simulink model "Vehicle_Model_Controller_2018"  (R2020a)
settings: Solver=FixedStepAuto  StartTime=0.0  StopTime=60  FixedStep=0.015  MaxStep=0.1  RelTol=1e-3
model workspace (MAT data in the model file):
  Kp = 10
  understeer_gradient = 0.05
undefined symbols (not defined in the file or in its folder): front_forces, rear_forces
libraries: fl_lib x24, nesl_utility x20, sdl_lib x8, simulink x1, vehdynlibsteering x1, autolibshared x1, autolibdatasheetbattery x1
(part 2 of 2)

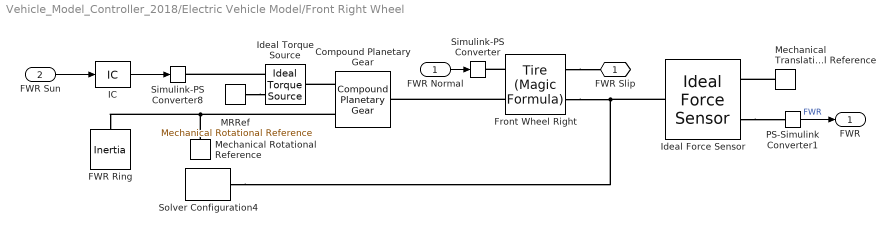
== system Vehicle_Model_Controller_2018/Electric Vehicle Model/Front Right Wheel ==
  FWR Normal : Inport
  FWR Sun : Inport  Port=2
  Compound Planetary Gear : sdl_lib/Gears/Compound Planetary Gear  rp_ratio=84/23  ps_ratio=37/24  friction_model=sdl.enum.gear_friction.none  mu_visc=[0, 0] N*m/(rad/s)  efficiency=[.96, .98]  temperature_TLU=[280, 300, 320] K  efficiency_sp_TLU=[.95, .9, .85]  efficiency_rp_TLU=[.95, .9, .85]  pwr_thr=[.001, .001] W  thermal_mass=50 J/K  T_init=300 K  model_inertia=simscape.enum.onoff.off  planet_inertia=0.001 kg*m^2
      settings: SourceProductBaseCode=LD  InternalSimscapePortConfiguration="{\"Bottom\":[],\"Left\":[{\"id\":\"C\",\"label\":\"C\",\"type\":\"foundation.mechanical.rotational.rotational\"}],\"Right\":[{\"id\":\"R\",\"label\":\"R\",\"type\":\"foundation.mechanical.rotational.rotational\"},{\"id\":\"S\",\"label\":\"S\",\"type\":\"foundation.mechanical.rotational.rotational\"}],\"Top\":[]}"
  FWR Ring : fl_lib/Mechanical/Rotational Elements/Inertia  inertia=0.1 kg*m^2  num_ports=foundation.enum.numPorts2.one  w_specify=off  w_priority=High  w=0 rad/s  w_nominal_specify=off  w_nominal_unit=rad/s  w_nominal_value=1  t_specify=off  t_priority=None  t=0 N*m  t_nominal_specify=off  t_nominal_unit=N*m  t_nominal_value=1
  Front Wheel Right : sdl_lib/Tires & Vehicles/Tire (Magic Formula)  parameterization=sdl.enum.magic_tire_model.peak  F_z1=3000 N  F_x1=3500 N  kappa1=10  B_m=10  C_m=1.9  D_m=1  E_m=0.97  fz0=4000 N  p_Cx=1.685  p_Dx=[1.21, -.037]  p_Ex=[.344, .095, -.02, 0]  p_Kx=[21.51, -.163, .245]  p_Hx=[-.002, .002]  p_Vx=[0, 0]  v_tr_thr=0.1 m/s  r_e=0.3 m  model_compliance=0  stiffness=2e5 N/m  damping=1000 N/(m/s)  model_inertia=0  inertia=0.03 kg*m^2  initial_velocity=0 rad/s  model_resistance=0  resistance_model=2  coeff=0.015  p_tire=250e3 Pa  alpha=-0.003  beta=0.97  coeff_a=84e-4  coeff_b=6.2e-4 s/m  coeff_c=1.6e-4 s^2/m^2  v_thr=0.001 m/s
  IC : InitialCondition  Value=0
  Ideal Force Sensor : fl_lib/Mechanical/Mechanical Sensors/Ideal Force Sensor
  Ideal Torque Source : fl_lib/Mechanical/Mechanical Sources/Ideal Torque Source
      settings: SourceProductName=Foundation Library
  MRRef : fl_lib/Mechanical/Rotational Elements/Mechanical Rotational Reference
      settings: SourceProductName=Foundation Library
  Mechanical Rotational Reference : fl_lib/Mechanical/Rotational Elements/Mechanical Rotational Reference
  Mechanical Translational Reference : fl_lib/Mechanical/Translational Elements/Mechanical Translational Reference
  PS-Simulink Converter1 : nesl_utility/PS-Simulink Converter  PhysicalDomain=network_engine_domain  SubClassName=ps_output  LeftPortType=input  RightPortType=output  PseudoPeriodic=off  Frequencies=[]  Unit=inherit  AffineConversion=off
      settings: SourceProductBaseCode=PW,SS
  Simulink-PS Converter : nesl_utility/Simulink-PS Converter  PhysicalDomain=network_engine_domain  SubClassName=ps_input  LeftPortType=input  RightPortType=output  PseudoPeriodic=off  Frequencies=[]  NoiseDistribution=none  NoiseParameters=[]  Unit=N  AffineConversion=off  FilteringAndDerivatives=zero  SimscapeFilterOrder=1  InputFilterTimeConstant=0.001  UdotUserProvided=0
      settings: SourceProductBaseCode=PW,SS
  Simulink-PS Converter8 : nesl_utility/Simulink-PS Converter  PhysicalDomain=network_engine_domain  SubClassName=ps_input  LeftPortType=input  RightPortType=output  PseudoPeriodic=off  Frequencies=[]  NoiseDistribution=none  NoiseParameters=[]  Unit=N*m  AffineConversion=off  FilteringAndDerivatives=zero  SimscapeFilterOrder=1  InputFilterTimeConstant=0.001  UdotUserProvided=0
      settings: SourceProductBaseCode=PW,SS
  Solver Configuration4 : nesl_utility/Solver Configuration  PhysicalDomain=network_engine_domain  SubClassName=solver  LeftPortType=input  RightPortType=generic  Tones=[]  Harmonics=[]  SimulateNoise=off  Profile=off  UseLocalSampling=off  EnableSwitchedLinearOptims=on  FrequencyDomain=off  UseCCode=off  RelTol=0.001  AbsTol=1e-06  MinStep=1e-09  ToWorkspace=off  RevertToSquareIcSolve=off  NumHomotopyIterations=100  PhasorMode=off  PhasorModeNumHarmonics=1  DoDC=on  ResidualTolerance=1e-09  UseLocalSolver=off  LocalSolverChoice=NE_BACKWARD_EULER_ADVANCER  LocalSolverSampleTime=0.001  DoFixedCost=off  MaxNonlinIter=3  MaxModeIter=2  ComputeImpulses=off  ImpulseIterations=2  LinearAlgebra=auto  EquationFormulation=NE_TIME_EF  DelaysMemoryBudget=1024  AutomaticFiltering=on  FilteringTimeConstant=0.001  PartitionStorageMethod=AS_NEEDED  PartitionMemoryBudget=1024  PartitionMethod=ROBUST
      settings: SourceProductBaseCode=PW,SS
  FWR Slip : PMIOPort  Side=Right
  FWR : Outport
  wires:
  PS-Simulink Converter1/1 -> FWR/1  "FWR"
  FWR Normal/1 -> Simulink-PS Converter/1
  IC/1 -> Simulink-PS Converter8/1
  FWR Sun/1 -> IC/1
  connections:
  Front Wheel Right/RConn1 -- FWR Slip/RConn1
  Front Wheel Right/LConn1 -- Simulink-PS Converter/RConn1
  Ideal Force Sensor/RConn2 -- PS-Simulink Converter1/LConn1
  Ideal Force Sensor/LConn1 -- Front Wheel Right/RConn2 -- Solver Configuration4/RConn1
  Mechanical Translational Reference/LConn1 -- Ideal Force Sensor/RConn1
  MRRef/LConn1 -- Ideal Torque Source/RConn2
  Compound Planetary Gear/RConn2 -- Ideal Torque Source/LConn1
  Ideal Torque Source/RConn1 -- Simulink-PS Converter8/RConn1
  Front Wheel Right/LConn2 -- Compound Planetary Gear/LConn1
  Mechanical Rotational Reference/LConn1 -- FWR Ring/LConn1 -- Compound Planetary Gear/RConn1

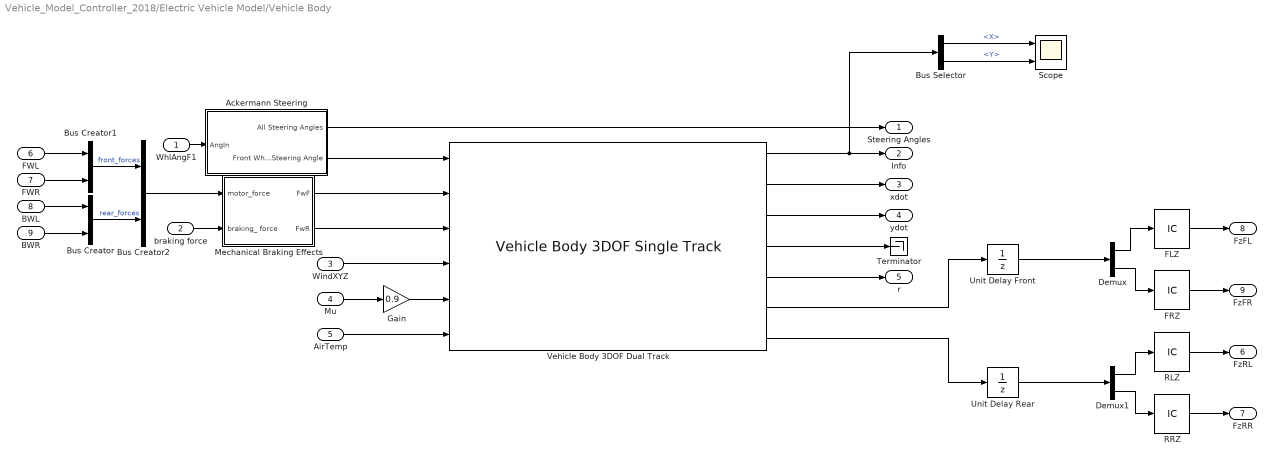
== system Vehicle_Model_Controller_2018/Electric Vehicle Model/Vehicle Body ==
  WhlAngF1 : Inport
  braking force : Inport  Port=2
  WindXYZ : Inport  Port=3
  Mu : Inport  Port=4
  AirTemp : Inport  Port=5
  FWL : Inport  Port=6
  FWR : Inport  Port=7
  BWL : Inport  Port=8
  BWR : Inport  Port=9
  Ackermann Steering : Subsystem
  Bus Creator : BusCreator  Inputs=BWL Force,BWR Force
  Bus Creator1 : BusCreator  Inputs=FWL Force,FWR Force
  Bus Creator2 : BusCreator  Inputs=front_forces,rear_forces
  Bus Selector : BusSelector  OutputSignals=InertFrm.Cg.Disp.X,InertFrm.Cg.Disp.Y
  Demux : Demux  Outputs=2
  Demux1 : Demux  Outputs=2
  FLZ : InitialCondition  Value=400
  FRZ : InitialCondition  Value=400
  Gain : Gain  Gain=0.9
  Mechanical Braking Effects : Subsystem
  RLZ : InitialCondition  Value=400
  RRZ : InitialCondition  Value=400
  Scope : Scope  NumInputPorts=2
  Terminator : Terminator
  Unit Delay Front : UnitDelay  SampleTime=-1  HasFrameUpgradeWarning=on
  Unit Delay Rear : UnitDelay  SampleTime=-1  HasFrameUpgradeWarning=on
  Vehicle Body 3DOF Dual Track : autolibshared/Vehicle Body 3DOF Single Track  trackMode=Dual  inputMode=External longitudinal forces  frontSteerMode=on  rearSteerMode=off  windMode=on  muMode=on  extFMode=off  extMMode=off  htchFMode=off  htchMMode=off  extXo=off  extpsio=off  extxdoto=off  extro=off  extYo=off  extTamb=on  extydoto=off  aMode=2  NF=2  NR=2  m=223  a=1  b=1  h=0.35  dh=1  hh=0.2  X_o=0  xdot_o=0  CalphaMode=off  sigmaMode=on  d=0  hl=0  w=[1.4,1.4]  Cy_f=12e3  Cy_r=11e3  sigma_f=.1  sigma_r=.1  alpha_f_brk=[-.1 .1]  Cy_f_data=[-9e3 9e3]  alpha_r_brk=[-.1 .1]  Cy_r_data=[-9e3 9e3]  Y_o=0  ydot_o=0  Izz=4000  psi_o=0  r_o=0  Af=1  Cd=.3  Cl=.1  Cpm=.1  beta_w=[0:0.01:0.3]  Cs=[0:0.03:0.9]  Cym=[0:0.01:0.3]  Pabs=101325  Tair=273  g=9.81  mu=1  xdot_tol=.1  Fznom=5000  Fxtire_sat=7e4  Fytire_sat=7e4  longOff=0  latOff=0  vertOff=0  wrapAng=off
      settings: SourceProductBaseCode=PW,MT,UV,VE,VP
  Steering Angles : Outport
  Info : Outport  Port=2
  xdot : Outport  Port=3
  ydot : Outport  Port=4
  r : Outport  Port=5
  FzRL : Outport  Port=6
  FzRR : Outport  Port=7
  FzFL : Outport  Port=8
  FzFR : Outport  Port=9
  wires:
  Vehicle Body 3DOF Dual Track/3 -> ydot/1
  Mechanical Braking Effects/1(FwF) -> Vehicle Body 3DOF Dual Track/2
  Vehicle Body 3DOF Dual Track/1 -> Info/1, Bus Selector/1
  Vehicle Body 3DOF Dual Track/2 -> xdot/1
  AirTemp/1 -> Vehicle Body 3DOF Dual Track/6
  Vehicle Body 3DOF Dual Track/4 -> Terminator/1
  Vehicle Body 3DOF Dual Track/5 -> r/1
  Mechanical Braking Effects/2(FwR) -> Vehicle Body 3DOF Dual Track/3
  Ackermann Steering/2(Front Wheels Steering Angle) -> Vehicle Body 3DOF Dual Track/1
  WindXYZ/1 -> Vehicle Body 3DOF Dual Track/4
  Unit Delay Front/1 -> Demux/1
  Vehicle Body 3DOF Dual Track/6 -> Unit Delay Front/1
  Demux/1 -> FLZ/1
  Demux/2 -> FRZ/1
  FLZ/1 -> FzFL/1
  FRZ/1 -> FzFR/1
  FWL/1 -> Bus Creator1/1
  FWR/1 -> Bus Creator1/2
  Unit Delay Rear/1 -> Demux1/1
  RLZ/1 -> FzRL/1
  RRZ/1 -> FzRR/1
  Demux1/1 -> RLZ/1
  Demux1/2 -> RRZ/1
  Vehicle Body 3DOF Dual Track/7 -> Unit Delay Rear/1
  BWL/1 -> Bus Creator/1
  BWR/1 -> Bus Creator/2
  Bus Creator2/1 -> Mechanical Braking Effects/1(motor_force)
  braking force/1 -> Mechanical Braking Effects/2(braking_	force)
  Bus Creator1/1 -> Bus Creator2/1  "front_forces"
  Bus Creator/1 -> Bus Creator2/2  "rear_forces"
  Gain/1 -> Vehicle Body 3DOF Dual Track/5
  Mu/1 -> Gain/1
  Ackermann Steering/1(All Steering Angles) -> Steering Angles/1
  WhlAngF1/1 -> Ackermann Steering/1(AngIn)
  Bus Selector/1 -> Scope/1  "<X>"
  Bus Selector/2 -> Scope/2  "<Y>"

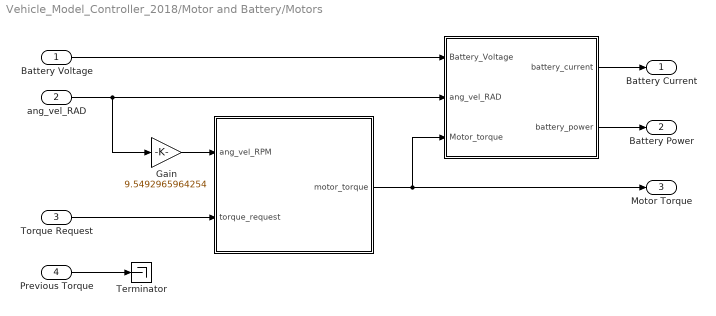
== system Vehicle_Model_Controller_2018/Motor and Battery/Motors ==
  Battery Voltage : Inport
  ang_vel_RAD : Inport  Port=2
  Torque Request : Inport  Port=3
  Previous Torque : Inport  Port=4
  " " : MATLAB Function  TreatAsAtomicUnit=on
  "  " : MATLAB Function  TreatAsAtomicUnit=on
  Gain : Gain  Gain=9.5492965964254
  Terminator : Terminator
  Battery Current : Outport
  Battery Power : Outport  Port=2
  Motor Torque : Outport  Port=3
  wires:
  Torque Request/1 -> " "/2(torque_request)
  Battery Voltage/1 -> "  "/1(Battery_Voltage)
  ang_vel_RAD/1 -> Gain/1, "  "/2(ang_vel_RAD)
  "  "/1(battery_current) -> Battery Current/1
  " "/1(motor_torque) -> Motor Torque/1, "  "/3(Motor_torque)
  "  "/2(battery_power) -> Battery Power/1
  Gain/1 -> " "/1(ang_vel_RPM)
  Previous Torque/1 -> Terminator/1

== system Vehicle_Model_Controller_2018/Electric Vehicle Model/Vehicle Body/Ackermann Steering ==
  AngIn : Inport
  Bus Creator : BusCreator  Inputs=2
  Deg to Rad : Gain  Gain=pi/180
  Kinematic Steering : vehdynlibsteering/Kinematic Steering  StrgType=Ackerman  StrgRatioType=Constant  Loc=Front  NrmlFctr=1  TrckWdth=1  WhlBase=1.524  Db=0  StrgRng=1.25*pi  StrgAngBpts="[-6.2832   -5.0265   -3.7699   -2.5133   -1.2566         0    1.2566    2.5133    3.7699    5.0265    6.2832]"  StrgRatioTbl=|  StrgRatio=1  StrgArmLngth=0.1  RckCsLngth=0.5  TieRodLngth=0.248  D=0.2  PnnRadius=0.0057  PnnRadiusTbl="[0.0055    0.0055    0.0056    0.0057    0.0058    0.0057    0.0057    0.0057    0.0056    0.0055    0.0055]"  RodLngth=0.1  ParaArmLngth=0.9  aMode=2
      | [13.5000   13.3750   13.2500   13.1250   13.0000   13.0000   13.0000   13.1250   13.2500   13.3750   13.5000
      | ]
  Mux3 : Mux  Inputs=2
  Terminator : Terminator
  All Steering Angles : Outport
  Front Wheels Steering Angle : Outport  Port=2
  wires:
  Kinematic Steering/2 -> Mux3/1
  Kinematic Steering/3 -> Mux3/2
  Kinematic Steering/1 -> Terminator/1
  Mux3/1 -> Front Wheels Steering Angle/1, Bus Creator/1  "ackermann angles"
  Bus Creator/1 -> All Steering Angles/1
  Deg to Rad/1 -> Kinematic Steering/1, Bus Creator/2  "steering_angle"
  AngIn/1 -> Deg to Rad/1  "steering_angle"

== system Vehicle_Model_Controller_2018/Electric Vehicle Model/Vehicle Body/Mechanical Braking Effects ==
  motor_force : Inport
  braking_	force : Inport  Port=2
  Bus Selector : BusSelector  OutputSignals=front_forces,rear_forces
  mechanical_braking_effects : MATLAB Function  TreatAsAtomicUnit=on
  FwF : Outport
  FwR : Outport  Port=2
  wires:
  mechanical_braking_effects/1(FwF) -> FwF/1
  braking_	force/1 -> mechanical_braking_effects/1(braking_forces)
  mechanical_braking_effects/2(FwR) -> FwR/1
  Bus Selector/1 -> mechanical_braking_effects/2(front_forces)  "<front_forces>"
  Bus Selector/2 -> mechanical_braking_effects/3(rear_forces)  "<rear_forces>"
  motor_force/1 -> Bus Selector/1

== matlab function Vehicle_Model_Controller_2018/Driver Input Logic/Torque Vectoring Controller/Layer 2 ==
  data: prev_torque input; yaw_err output; J_z output; T_F input; P_L input; eff_m input; s input; yaw_ref input; yaw input; J_z input; l input; a_theta input; c_theta input; F_I input; P_A input; vel input; Fy input; gr input; r input; F_max input; y output; x output; Fy_wheel output; F_I output; P_A output; eff_m output; T_F output; slip_limit output; power_limit output; omega_m output size=[1 4]; t_upper output; tau input; t_minmax input; t_lower output; f input
function [yaw_err, J_z, y, x, Fy_wheel, F_I, P_A, eff_m, T_F, slip_limit, power_limit, omega_m, t_upper, t_lower] = Layer_2(prev_torque, T_F, P_L, eff_m, s, yaw_ref, yaw, J_z, l, a_theta, c_theta, F_I, P_A, vel, Fy, gr, r, F_max, tau, t_minmax, f)
%% Calculations
% Calculate the Yaw Error, Apply Sign Convention
if yaw_ref(1) == 0 && yaw(1) == 0
    yaw_err = 0;
elseif c_theta >= 0
    yaw_err = min(abs(yaw_ref)) - yaw;
else
    yaw_err = (min(abs(yaw_ref)) * -1) - yaw;
end


% Motor Shaft Speed, RAD/S
omega_fl = sqrt((vel(1) * cos(a_theta(1)))^2 + (vel(2) * sin(a_theta(1)))^2);
omega_fr = sqrt((vel(3) * cos(a_theta(2)))^2 + (vel(4) * sin(a_theta(2)))^2);
omega_rl = vel(5);
omega_rr = vel(6);

omega_m = [omega_fl, omega_fr, omega_rl, omega_rr] .* (gr ./ r);


% Calculate K_1 Vehicle Constants
x_1 = (s(1) * cos(a_theta(1))) + (l(1) * sin(a_theta(1)));    
x_2 = (-1 * s(1) * cos(a_theta(2))) + (l(1) * sin(a_theta(2)));     
x_3 = s(2);     
x_4 = -s(2); 

x = [x_1, x_2, x_3, x_4]; 


% Transform Lateral Forces (Vehicle) to Lateral Forces (Wheel)
F_y_ij_fl = (sin(a_theta(1)) * Fy(1)) + (cos(a_theta(1)) * Fy(1));
F_y_ij_fr = (sin(a_theta(2)) * Fy(2)) + (cos(a_theta(2)) * Fy(2));
F_y_ij_rl = Fy(3);
F_y_ij_rr = Fy(4);

Fy_wheel = [F_y_ij_fl, F_y_ij_fr, F_y_ij_rl, F_y_ij_rr];


% Calculate K_2 Vehicle Constants
y_1 = (-1 * s(1) * sin(a_theta(1))) + (l(1) * cos(a_theta(1)));    
y_2 = (s(1) * sin(a_theta(2))) + (l(1) * cos(a_theta(2)));
y_3 = -l(2);
y_4 = -l(2);

y = [y_1, y_2, y_3, y_4]; 


% Torque Limits On Individual Wheels
Fx_max2 = (F_max.^2)-(Fy_wheel.^2);

% Control For Negative Output
for i = 1:4
    if Fx_max2(i) < 0
        Fx_max2(i) = 0;
    end
end

% Calculate Torque Limit Due to Power and Slip
Fx_max = sqrt(Fx_max2);
slip_limit = Fx_max ./ T_F; 
power_limit = (P_L .* eff_m) ./ omega_m;

% Erase power limit solution above torque limit, for better data
% visualization
for i = 1:4
    if power_limit(i) > 25
        power_limit(i) = 25;
    end
end 

% Calculate Constants for getting limit on motor output torque
e_term = exp(-1 / (tau * f));
c_lower = (1 - e_term) .* t_minmax(1);
c_upper = (1 - e_term) .* t_minmax(2);
c_constant = (prev_torque .* e_term)';

% Max and Min Torque Limits
t_upper = max([c_upper + c_constant; c_constant + .01]);
t_lower = min([c_lower + c_constant; c_constant - .01]);


end

== matlab function Vehicle_Model_Controller_2018/Motor and Battery/Motors/  ==
  data: ang_vel_RPM input; motor_torque output size=[1 4]; torque_request input
function motor_torque = get_torque(ang_vel_RPM, torque_request)
%% Actual Torque Output
% Developers:    Demetrius Gulewicz

% Developed for: Purdue Electric Racing
% Date:          09/18/2021
%
% Definitions:
% ang_vel:   Angular velocity of each wheel on the wheel fixed y axis [RPM]
% torque_request: Requested torque from the LP model                  [Nm]

%% Constants
% quadratic constants that connect current and max RPM of motors
a_v = 0.2667;
b_v = -66.353;
c_v = 10452 - ang_vel_RPM;

% quadratic constants that connnect current and max torque of motors
a_t = -0.0987;
b_t = 45.799;
c_t = -129.65;

% maximum possible current at the current RPM
max_current = [0, 0, 0, 0];


%% Calculate Maximum Torque Possible
% calculate the maximum current possible at the current RPM
for i = [1:4]
   if ang_vel_RPM(i) < 7000
       max_current(i) = 70;
   else
       max_current(i) = (-b_v - sqrt(b_v^2 - (4*a_v.*c_v(i)))) .* (1/(2*a_v));
   end
end

% calculate the meximum torque at the max current
max_torque = (a_t .* (max_current.^2)) + (b_t .* max_current) + c_t;
for i = [1:4]
   if max_torque(i) < 0
      max_torque(i) = 0;
   end
end

motor_torque_matrix = [max_torque; torque_request'];
motor_torque = min(motor_torque_matrix);

== matlab function Vehicle_Model_Controller_2018/Electric Vehicle Model/Vehicle Body/Mechanical Braking Effects/mechanical_braking_effects ==
  data: braking_forces input; front_forces input; FwF output; rear_forces input; FwR output
function [FwF, FwR] = Mechanical_Braking_Effects(braking_forces, front_forces, rear_forces)
%% Mechanical Braking Effects
% Developers:    Demetrius Gulewicz
% Developed for: Purdue Electric Racing
% Date:          09/01/2021
%
% Definitions:
% front_force:      force vector from the front motors    [N]
% braking_forces:   braking force vector on all 4 tires   [N]
% rear_forces:      force vector from the rear motors     [N]

%% Calculation
FwF = front_forces - braking_forces(1:2);
FwR = rear_forces - braking_forces(3:4);

== matlab function Vehicle_Model_Controller_2018/Driver Input Logic/Braking Controller/MATLAB Function ==
  data: driver_input input; T_x_ij output double
function T_x_ij = split_braking_torque(driver_input)
%% Regenerative Braking Force Split
% Developers:    Demetrius Gulewicz
% Developed for: Purdue Electric Racing
% Date:          09/01/2021
%
% Definitions:
% driver_input:   sum of forces requested by driver to the 4 motors   [N]
%% Constants
R = 0.3;        % wheel radius                              [m]


%% Calculation
driver_torque = (driver_input * R)/ 4;


T_x_ij = [driver_torque; driver_torque; driver_torque; driver_torque];

== matlab function Vehicle_Model_Controller_2018/Driver Input Logic/Torque Vectoring Controller/LP_Calc  ==
  data: Tx output size=[4 1]; omega_m output; lb output double; PID input; J_z input; y input; x input; Fy_wheel input; F_I input; P_A input; eff_m input; T_F input; slip_limit input; power_limit input; omega_m input; t_upper input; ub output double; A output double; b output double; Aeq output double; beq output double; t_lower input
function [Tx, omega_m, lb, ub, A, b, Aeq, beq] = LP_calc(PID, J_z, y, x, Fy_wheel, F_I, P_A, eff_m, T_F, slip_limit, power_limit, omega_m, t_upper, t_lower)
%% Calculation
% Calculate Boundary Conditions
ub = [0, 0, 0, 0];
lb = [0, 0, 0, 0];

for i = 1:4
    ub(i) = min([slip_limit(i), power_limit(i), 20, t_upper(i)]);
    lb(i) = max(-1 * ub(i), t_lower(i));
end

% Calculate Yaw Constraint
Aeq = ((1 ./ J_z) .* x) .* T_F;
beq = PID-sum(((1 / J_z) * y) .* Fy_wheel);

% Calculate User Requested Torque Limit
A = omega_m ./ eff_m;
b = F_I * P_A;


%% Optimization
% Set Initial Guess
x0 = [5, 5, 5, 5];

% Set Optimization Parameters
options = optimoptions('fmincon','Algorithm','sqp');

% Maximize the Forces Acting on the Car
objfun = @(x) -(x(1) * T_F(1))-(x(2) * T_F(2))-(x(3) * T_F(3))-(x(4) * T_F(4));

% Find the Optimal Solution
Tx = fmincon(objfun,x0,A,b,Aeq,beq,lb,ub,[],options)';

end

== matlab function Vehicle_Model_Controller_2018/Motor and Battery/Motors/   ==
  data: Battery_Voltage input; ang_vel_RAD input; battery_current output; Motor_torque input; battery_power output
function [battery_current, battery_power]= get_batt_curr(Battery_Voltage, ang_vel_RAD, Motor_torque)
%% Current Draw
% Developers:    Demetrius Gulewicz

% Developed for: Purdue Electric Racing
% Date:          09/18/2021
%
% Definitions:
% ang_vel_RAD:   Angular velocity of each wheel on the wheel fixed y axis [RAD]
% Motor_torque:  Torque the motor actually outputs                 [Ncm]
% Battery_Voltage: The voltage of the battery                      [V]

%% Definitions
a = 0.0411;
b = 2.7976;
c = 45.978;

t = Motor_torque;
w = ang_vel_RAD;
v = Battery_Voltage;

e = 85;

%% Calculate Current Draw
%x0 = [20, 20, 20, 20];
%options = optimoptions('fsolve','Algorithm','Levenberg-Marquardt');
%F = @(x) ([(a * x(1)^3) + (b * x(1)^2) + (c * x(1)), ] .* v) - (t .* w);
%battery_current = sum(fsolve(F,x0,options));

battery_current = sum((t .* w') ./ (e .* v));
battery_power = battery_current * Battery_Voltage;
end

== matlab function Vehicle_Model_Controller_2018/Driver Input Logic/Torque Vectoring Controller/Constants  ==
  data: P_L output; C_L output; eff_m output; mu output; g output; buff output; r output; s output; l output; J_z output; K_u output; gr output; eff_g output; tau output; t_minmax output; f output
function [P_L, C_L, eff_m, mu, g, buff, r, s, l, J_z, K_u, gr, eff_g, tau, t_minmax, f] = def_c()
%% Define Constants
% General Constants
mu = [1, 1, 1, 1]; % Maximum friction coefficient [Unitless]
g = 9.81; % Gravitational constant [m/s^2]
buff = 0.05; % Buffer value when calculating max allowable yaw
f = 30; % controller runtime frequency [Hz]

% Motor Constants
P_L = [15, 15, 15, 15] * 1000; % Power limit for each motor [W] 
C_L = [70, 70, 70, 70]; % Current limit for each motor [Amp]
eff_m = [0.85, 0.85, 0.85, 0.85]; % Motor efficiency [Unitless]
tau = 0.09; % Motor Response Time Constant
t_minmax = [-25, 25]; % Minimum and maximum torque you can request from motor

% General Vehicle Constants
r = 0.3; % Tire radius [m]
s = [1, 1]; % Half track width [m]
l = [1, 1]; % Wheelbase [m]
J_z = 4000; % Polar moment of inertia [kg m^2]
K_u = 0.05; % Understeer gradient

% Gearbox Constants
GR_f = (37/24) * (84/23) + 1; % Front gear ratio [Unitless]
GR_r = (40/21) * (84/23) + 1; % Rear gear ratio [Unitless]
gr = [GR_f, GR_f, GR_r, GR_r]; % Gear ratios [Unitless]
eff_g = 0.97; % Gearbox power transmission efficiency [Unitless]


end

== matlab function Vehicle_Model_Controller_2018/Driver Input Logic/Torque Vectoring Controller/Layer 1 ==
  data: T_F output; P_L output; eff_m output; s output; yaw_ref output; yaw output; J_z output; l output; a_theta output; c_theta output; F_I output; P_A output; vel output; Fy output; gr output; r output; F_max output; P_L input; C_L input; eff_m input; mu input; g input; buff input; r input; s input; l input; J_z input; K_u input; gr input; eff_g input; tau input; t_minmax input; f input; F_I input; P_A input; c_theta input; a_theta input; Fx input; Fy input; Fz input; Vx input; Vy input; yaw input; vel input; tau output; t_minmax output; f output
function [T_F, P_L, eff_m, s, yaw_ref, yaw, J_z, l, a_theta, c_theta, F_I, P_A, vel, Fy, gr, r, F_max, tau, t_minmax, f] = Layer_1(P_L, C_L, eff_m, mu, g, buff, r, s, l, J_z, K_u, gr, eff_g, tau, t_minmax, f, F_I, P_A, c_theta, a_theta, Fx, Fy, Fz, Vx, Vy, yaw, vel)
%% Calculation
% Max Allowed Force On Each Wheel
F_max = abs(mu'.*Fz)';

% Convert Torque At The Motor Shaft to Force At The Wheel
T_F = (gr .* eff_g) ./ r;


% Yaw Calculations
v_cog = sqrt(Vx^2 + Vy^2);
yaw_des = (v_cog * abs(c_theta)) / ((l(1) + l(2)) + (K_u * v_cog ^ 2));
yaw_max = (max(mu) * g) / (v_cog + buff);
yaw_ref = [yaw_des, yaw_max];

end
